simulink model "snap2_f_200msps_64i_4096c"  (R2019a)
settings: Solver=VariableStepDiscrete  StartTime=0.0  StopTime=10.0  RelTol=1e-3
undefined symbols (not defined in the file or in its folder): datetime, posixtime
libraries: xbsIndex_r4 x21354, casper_library_misc x297, casper_library_delays x19, xps_library x14, casper_library_sources x4
(part 13 of 217)

== system snap2_f_200msps_64i_4096c/cosmic_ray/Subsystem1 ==
  Constant24 : xbsIndex_r4/Constant  const=1  gui_display_data_type=Boolean  arith_type=Boolean  n_bits=1  bin_pt=0  preci_type=Single  exp_width=8  frac_width=24  explicit_period=on  period=1  equ=P=C  opselect=C  inp2=PCIN>>17  opr=+  inp1=P  carry=CIN  dbl_ovrd=off  block_type=constant
  Convert5 : xbsIndex_r4/Convert  gui_display_data_type=Boolean  arith_type=Boolean  n_bits=16  bin_pt=14  float_type=Single  exp_bits=8  fraction_bits=24  quantization=Truncate  overflow=Wrap  en=off  latency=1  pipeline=off  dbl_ovrd=off  block_type=convert
  Delay15 : xbsIndex_r4/Delay  rst=off  infoeditControl=Selection of Reset will increase slice count due to use of real FFs and instead of SRLs  en=off  latency=5000  reg_retiming=on  dbl_ovrd=off  block_type=delay
  Inverter5 : xbsIndex_r4/Inverter  en=off  latency=1  dbl_ovrd=off  block_type=inv
  Logical6 : xbsIndex_r4/Logical  logical_function=AND  inputs=2  en=off  latency=1  precision=Full  arith_type=Unsigned  n_bits=16  bin_pt=0  align_bp=on  dbl_ovrd=off  block_type=logical
  Slice22 : xbsIndex_r4/Slice  nbits=1  boolean_output=off  mode=Upper Bit Location + Width  bit1=0  base1=MSB of Input  bit0=0  base0=LSB of Input  dbl_ovrd=off  block_type=slice
  edge_detect4 : Subsystem  AncestorBlock=casper_library_misc/edge_detect  mask(edge_detect){edge=Rising, polarity=Active High, x_in=[0 0.08 0.08 0.16 0.16 0.24 0.24 0.32 0.32 0.4], y_in=[-1 -1  1  1  1  1  1  1  1  1], x_out=[0.6 0.68 0.68 0.76 0.76 0.84 0.84 0.92 0.92 1], y_out=[-1 -1  1  1 -1 -1 -1 -1 -1 -1]}
      mask prompts: edge "Edge Type"; polarity "Output Polarity"; x_in "Input X Positions"; y_in "Input Y Positions"; x_out "Output X Positions"; y_out "Output Y Positions"
      mask help: Output is active for one-cycle after each edge of the specified type (i.e. rising, falling or both).
      mask init: same as snap2_f_200msps_64i_4096c/cosmic_ray/edge_detect
      settings: AttributesFormatString=|
      | rising edges
      | active high
      mask Help: Output is active for one-cycle after each edge of the specified type (i.e. rising, falling, or both).  Latency is zero.
      mask TypeOptions edge: Rising | Falling | Both
      mask TypeOptions polarity: Active High | Active Low
      mask Display:
      | plot(x_in_num,0.5+y_in_num*0.2);
      | plot(x_out_num,0.5+y_out_num*0.2);
  trigger_sim5 : xbsIndex_r4/Counter  cnt_type=Free Running  cnt_to=1  operation=Up  start_count=1  cnt_by_val=1  arith_type=Unsigned  n_bits=3  bin_pt=0  load_pin=off  rst=off  en=on  explicit_period=off  period=1  use_behavioral_HDL=off  implementation=Fabric  dbl_ovrd=off  block_type=counter
  Out1 : Outport
  wires:
  Convert5/1 -> edge_detect4/1(in), Inverter5/1
  Slice22/1 -> Convert5/1
  Constant24/1 -> Logical6/2
  Delay15/1 -> Out1/1
  trigger_sim5/1 -> Slice22/1
  Logical6/1 -> trigger_sim5/1
  Inverter5/1 -> Logical6/1
  edge_detect4/1(out) -> Delay15/1

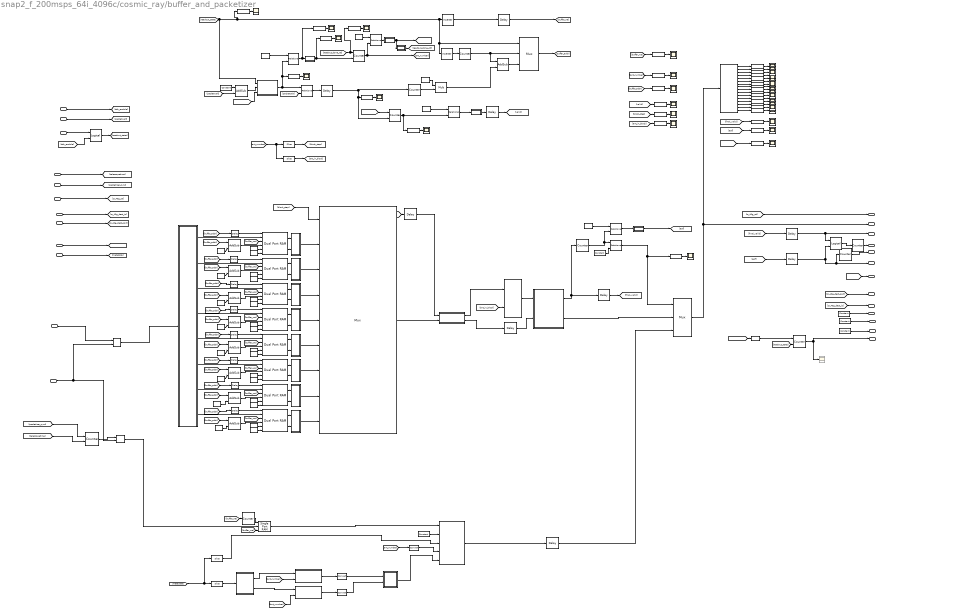
== system snap2_f_200msps_64i_4096c/cosmic_ray/buffer_and_packetizer ==
  note: The buffers' input is delayed is delayed in order to position the pulse in the middle of the buffer. The timestamp and data are delayed by the same amount.
  note: When load goes high, the counter takes the value provided by din, and then resumes counting up from there. Telescopetime is from tt_sync from the main design, which is the time of the last system sync expressed as unix time in number of clock cycles.
  note: Some delay here is needed to account for the time it takes the data to go through the rest of the packetizer. Probably a shorter delay around 20 clock cycles would suffice, but since the header only changes between packets, there shouldn't be any problem making it longer to be safe.
  note: The antenna counter increments whenever the main packet cycle counter falls back to zero. The readout is finished when the 6 bit antenna counter falls back to zero. Note that the last packet will be sent some (probably ~16) clock cycles after the readout done signal goes to 1, because it takes some time for the last data that is already on the way to make it through the packetizer.
  note: Note this works well in this situation where enable is high for a block of consecutive clock cycles. In other situations, it might have a limit that is up to 2 cycles lower. (So if copying this block to another design, test it).
  note: EOF and Valid both have a delay for the last mux on the data.
  note: 3 delay for counter, comparator and edge dectect above.
  note: Delay of 3 to account for buffer, mux, and delay on buffer address.
  note: 3 delays for valid to sync with buffer_addr during readout.
  note: Valid happens every 8 clock cycles.
  note: This counts to 2048 not 4096 because the address will increment in steps of two and both ports will be used to read out the buffer twice as fast as it was written.
  note: Data is buffered in dual-port BRAMs. Each of 8 BRAMS buffers 8 antennas bussed together. When writing data, the port A address continuesly increments by one on every clock cycle, as a circular buffer. Data input to port B is never enabled. When reading out data, both ports are used. Both addresses increment in steps of 2 and one port reads out odd time samples while the other reads out even samples. Both outputs are bussed together in order for the demux block to select the block of antennas that is currently being packetized.
  note: This block debusses the buffer output and then busses together adjacent pairs of samples from the same antenna and then does an 8x8 square transpose whose output on each clock cycle is 8 pairs of samples (total 16 consecutive samples) for one antenna. Every successive clock cycle is the next antenna, with the antenna repeating every 8 clock cycles.
  note: This mux increments which block of antennas to read out.
  note: Every valid increments the counter, which counts how many words have gone into the packet. Whenever the 8-bit counter loops back to zero, the packet header is inserted by the last mux below.
  note: End of frame occurs when the word counter resets.
  note: This mux chooses whether to send data or the header. The header is sent whenever the word count is zero-- i.e. the first word of the packet.
  note: Number of clock cycles spent in readout state.
  note: Signals that are only needed if receiving ethernet packets and thus are tied to zero in this design.
  note: Specifies the destination port and is controlled by a software register.
  note: Counters to track the number of eofs and eof+valid (which should be the number of packets). Eof must always occur on the last clock cycle where valid=1 for that packet, and so the eof counter and the eof+valid counter should match. Both are included for debugging purposes, as a common reason for not getting packets is when eof and valid misalign.
  note: Reset the ethernet port. This is tied to a software register.
  note: Data entering the ethernet block on clock cycles when valid=1 will go in the current packet.
  note: Data that will be clocked into the ethernet block whenever valid=1.
  note: End of frame to signify to the ethernet block that that the packet is ready.
  note: Readout is finished when eof occurs and the antenna number is 63.
  note: This is the packet header.
  note: convert to 8
  note: 3b
  note: 64b
  note: The timestamp buffer is write enabled whenever the data buffer is, but instead of reading out the whole timestamp buffer as is done for the data, the timestamp address stays fixed during readout at the place that it stopped writing. DOES THIS MEAN THAT THE TRANSMITTED TIMESTAMP IS THE OLDEST OR NEWEST IN THE BUFFER? It will be important to verify that the buffer address stops and restarts at the same address, and that this address is the same for the timestamp buffer and the data buffers.
  note: The upper three bits of the antenna number determine which block of 8 antennas is being packetized and the lower three bits determine which antenna within the block. These should increment during the wait between packets, so that the exact synchronization is less strict. However, if the delay through the other parts of the system is longer than packetwait, more careful delays on these signals may be needed.
  note: Wait for the software-tunable time between packets and then readout the buffer by cycling through addresses in steps of two, with odd and even being read out on the two different ports.
  note: Increment the buffer address by 1 whenever not in readout state, and by 2 when it's time to read out the buffer.
  note: Enable writing to the buffer whenever not in readout state. The delay of 3 is to sync up with the address when in listening state.
  note: Info to go in the packets saying if the trigger originated on this board, giving the board id, and saving the settings for the thresholds, windows, and roles.
  note: Counter number of clock cycles that the board spends in readout state during readout.
  note: Enable the timer while the board is in readout_state, reset from software.
  note: Specifies the destination ip and is controlled by a software register.
  note: This mux increments which antenna within the current block of antennas to read out. Out of the transpose block, every antenna repeats every 8 clock cycles. Single-antenna packets will be made by clocking data into the ethernet buffer once every 8 cycles. The choice of antenna is made by choosing between 8 different delay offsets on the sync signal, such that the valid is delayed according to which is chosen.
  pkt_wait : Inport
  tt : Inport  Port=2
  sync_in : Inport  Port=3
  eth40g_rst : Inport  Port=4
  dest_ip : Inport  Port=5
  dest_port : Inport  Port=6
  readout_timer_rst : Inport  Port=7
  data_in : Inport  Port=8
  readout_state : Inport  Port=9
  eth_enable : Inport  Port=10
  metadata : Inport  Port=11
  delay_buffer : Inport  Port=12
  AddSub : xbsIndex_r4/AddSub  mode=Addition  use_carryin=off  use_carryout=off  en=off  latency=1  precision=Full  arith_type=Unsigned  n_bits=16  bin_pt=14  quantization=Truncate  overflow=Wrap  use_behavioral_HDL=off  hw_selection=Fabric  pipelined=off  dbl_ovrd=off  block_type=addsub
  AddSub{1..9} (9 alike) : xbsIndex_r4/AddSub  mode=Addition  use_carryin=off  use_carryout=off  en=off  latency=1  precision=User Defined  arith_type=Unsigned  n_bits=12  bin_pt=0  quantization=Truncate  overflow=Wrap  use_behavioral_HDL=off  hw_selection=Fabric  pipelined=off  dbl_ovrd=off  block_type=addsub
  Constant : xbsIndex_r4/Constant  const=0  gui_display_data_type=Fixed-point  arith_type=Signed (2's comp)  n_bits=40  bin_pt=0  preci_type=Single  exp_width=8  frac_width=24  explicit_period=off  period=1  equ=P=C  opselect=C  inp2=PCIN>>17  opr=+  inp1=P  carry=CIN  dbl_ovrd=off  block_type=constant
  Constant{1,3..4,25} (4 alike) : xbsIndex_r4/Constant  const=0  gui_display_data_type=Fixed-point  arith_type=Unsigned  n_bits=3  bin_pt=0  preci_type=Single  exp_width=8  frac_width=24  explicit_period=on  period=1  equ=P=C  opselect=C  inp2=PCIN>>17  opr=+  inp1=P  carry=CIN  dbl_ovrd=off  block_type=constant
  Constant{6,8,10,12,14,16,18,20} (8 alike) : xbsIndex_r4/Constant  const=0  gui_display_data_type=Fixed-point  arith_type=Unsigned  n_bits=80  bin_pt=0  preci_type=Single  exp_width=8  frac_width=24  explicit_period=on  period=1  equ=P=C  opselect=C  inp2=PCIN>>17  opr=+  inp1=P  carry=CIN  dbl_ovrd=off  block_type=constant
  Constant{7,9,11,13,15,17,19,21} (8 alike) : xbsIndex_r4/Constant  const=0  gui_display_data_type=Boolean  arith_type=Boolean  n_bits=1  bin_pt=0  preci_type=Single  exp_width=8  frac_width=24  explicit_period=on  period=1  equ=P=C  opselect=C  inp2=PCIN>>17  opr=+  inp1=P  carry=CIN  dbl_ovrd=off  block_type=constant
  Constant{2,26..27,29..32,34} (8 alike) : xbsIndex_r4/Constant  const=1  gui_display_data_type=Fixed-point  arith_type=Unsigned  n_bits=1  bin_pt=0  preci_type=Single  exp_width=8  frac_width=24  explicit_period=on  period=1  equ=P=C  opselect=C  inp2=PCIN>>17  opr=+  inp1=P  carry=CIN  dbl_ovrd=off  block_type=constant
  Constant22 : xbsIndex_r4/Constant  const=0  gui_display_data_type=Boolean  arith_type=Boolean  n_bits=16  bin_pt=14  preci_type=Single  exp_width=8  frac_width=24  explicit_period=on  period=1  equ=P=C  opselect=C  inp2=PCIN>>17  opr=+  inp1=P  carry=CIN  dbl_ovrd=off  block_type=constant
  Constant23 : xbsIndex_r4/Constant  const=0  gui_display_data_type=Boolean  arith_type=Boolean  n_bits=16  bin_pt=14  preci_type=Single  exp_width=8  frac_width=24  explicit_period=on  period=1  equ=P=C  opselect=C  inp2=PCIN>>17  opr=+  inp1=P  carry=CIN  dbl_ovrd=off  block_type=constant
  Constant24 : xbsIndex_r4/Constant  const=2  gui_display_data_type=Fixed-point  arith_type=Unsigned  n_bits=2  bin_pt=0  preci_type=Single  exp_width=8  frac_width=24  explicit_period=on  period=1  equ=P=C  opselect=C  inp2=PCIN>>17  opr=+  inp1=P  carry=CIN  dbl_ovrd=off  block_type=constant
  Constant28 : xbsIndex_r4/Constant  const=0  gui_display_data_type=Boolean  arith_type=Boolean  n_bits=16  bin_pt=14  preci_type=Single  exp_width=8  frac_width=24  explicit_period=on  period=1  equ=P=C  opselect=C  inp2=PCIN>>17  opr=+  inp1=P  carry=CIN  dbl_ovrd=off  block_type=constant
  Constant33 : xbsIndex_r4/Constant  const=2048  gui_display_data_type=Fixed-point  arith_type=Unsigned  n_bits=12  bin_pt=0  preci_type=Single  exp_width=8  frac_width=24  explicit_period=on  period=1  equ=P=C  opselect=C  inp2=PCIN>>17  opr=+  inp1=P  carry=CIN  dbl_ovrd=off  block_type=constant
  Constant5 : xbsIndex_r4/Constant  const=0  gui_display_data_type=Fixed-point  arith_type=Unsigned  n_bits=8  bin_pt=0  preci_type=Single  exp_width=8  frac_width=24  explicit_period=on  period=1  equ=P=C  opselect=C  inp2=PCIN>>17  opr=+  inp1=P  carry=CIN  dbl_ovrd=off  block_type=constant
  Convert1 : xbsIndex_r4/Convert  gui_display_data_type=Fixed-point  arith_type=Unsigned  n_bits=8  bin_pt=0  float_type=Single  exp_bits=8  fraction_bits=24  quantization=Truncate  overflow=Wrap  en=off  latency=1  pipeline=off  dbl_ovrd=off  block_type=convert
  Convert2 : xbsIndex_r4/Convert  gui_display_data_type=Fixed-point  arith_type=Unsigned  n_bits=8  bin_pt=0  float_type=Single  exp_bits=8  fraction_bits=24  quantization=Truncate  overflow=Wrap  en=off  latency=1  pipeline=off  dbl_ovrd=off  block_type=convert
  Convert3 : xbsIndex_r4/Convert  gui_display_data_type=Fixed-point  arith_type=Unsigned  n_bits=8  bin_pt=0  float_type=Single  exp_bits=8  fraction_bits=24  quantization=Truncate  overflow=Wrap  en=off  latency=1  pipeline=off  dbl_ovrd=off  block_type=convert
  Counter2 : xbsIndex_r4/Counter  cnt_type=Free Running  cnt_to=Inf  operation=Up  start_count=0  cnt_by_val=1  arith_type=Unsigned  n_bits=32  bin_pt=0  load_pin=off  rst=off  en=on  explicit_period=on  period=1  use_behavioral_HDL=off  implementation=Fabric  dbl_ovrd=off  block_type=counter
  Counter5 : xbsIndex_r4/Counter  cnt_type=Free Running  cnt_to=Inf  operation=Up  start_count=0  cnt_by_val=1  arith_type=Unsigned  n_bits=32  bin_pt=0  load_pin=off  rst=off  en=on  explicit_period=on  period=1  use_behavioral_HDL=off  implementation=Fabric  dbl_ovrd=off  block_type=counter
  Delay1 : xbsIndex_r4/Delay  rst=off  infoeditControl=Selection of Reset will increase slice count due to use of real FFs and instead of SRLs  en=off  latency=3  reg_retiming=off  dbl_ovrd=off  block_type=delay
  Delay{2,4..10,12,14,16} (11 alike) : xbsIndex_r4/Delay  rst=off  infoeditControl=Selection of Reset will increase slice count due to use of real FFs and instead of SRLs  en=off  latency=1  reg_retiming=off  dbl_ovrd=off  block_type=delay
  Delay11 : xbsIndex_r4/Delay  rst=off  infoeditControl=Selection of Reset will increase slice count due to use of real FFs and instead of SRLs  en=off  latency=3  reg_retiming=off  dbl_ovrd=off  block_type=delay
  Delay13 : xbsIndex_r4/Delay  rst=off  infoeditControl=Selection of Reset will increase slice count due to use of real FFs and instead of SRLs  en=off  latency=2  reg_retiming=off  dbl_ovrd=off  block_type=delay
  Delay17 : xbsIndex_r4/Delay  rst=off  infoeditControl=Selection of Reset will increase slice count due to use of real FFs and instead of SRLs  en=off  latency=128  reg_retiming=off  dbl_ovrd=off  block_type=delay
  Delay24 : xbsIndex_r4/Delay  rst=off  infoeditControl=Selection of Reset will increase slice count due to use of real FFs and instead of SRLs  en=off  latency=1  reg_retiming=on  dbl_ovrd=off  block_type=delay
  Delay3 : xbsIndex_r4/Delay  rst=off  infoeditControl=Selection of Reset will increase slice count due to use of real FFs and instead of SRLs  en=off  latency=3  reg_retiming=off  dbl_ovrd=off  block_type=delay
  Dual Port RAM{,1..7} (8 alike) : xbsIndex_r4/Dual Port RAM  depth=4096  initVector=sin(pi*(0:15)/16)  distributed_mem=Block RAM  init_a=0  init_b=0  rst_a=off  rst_b=off  en_a=off  en_b=off  latency=1  write_mode_A=Read After Write  write_mode_B=Read After Write  optimize=Area  dbl_ovrd=off  block_type=dpram
  Gateway Out{2..34} (33 alike) : xbsIndex_r4/Gateway Out  inherit_from_input=off  hdl_port=on  rows=1  columns=1  UseAsDAC=off  DACChannel='1'  interface=None  automatic_assignment=on  address_offset=hex2dec('00')  intf_name=''  intf_description=''  timing_constraint=None  locs_specified=off  LOCs={}  io_standard={}  block_type=gatewayout
  Inverter : xbsIndex_r4/Inverter  en=off  latency=1  dbl_ovrd=off  block_type=inv
  Inverter1 : xbsIndex_r4/Inverter  en=off  latency=1  dbl_ovrd=off  block_type=inv
  Logical : xbsIndex_r4/Logical  logical_function=AND  inputs=2  en=off  latency=1  precision=Full  arith_type=Unsigned  n_bits=16  bin_pt=0  align_bp=on  dbl_ovrd=off  block_type=logical
  Logical3 : xbsIndex_r4/Logical  logical_function=AND  inputs=2  en=off  latency=1  precision=Full  arith_type=Unsigned  n_bits=16  bin_pt=0  align_bp=on  dbl_ovrd=off  block_type=logical
  Mult : xbsIndex_r4/Mult  precision=Full  arith_type="Signed  (2's comp)"  n_bits=16  bin_pt=14  quantization=Truncate  overflow=Wrap  en=off  latency=3  use_behavioral_HDL=off  opt=Speed  use_embedded=on  optimum_pipeline=off  pipeline=on  dbl_ovrd=off  use_rpm=on  placement_style=Triangular  block_type=mult
  Mux1 : xbsIndex_r4/Mux  inputs=2  en=off  latency=1  precision=Full  arith_type=Unsigned  n_bits=16  bin_pt=14  quantization=Truncate  overflow=Wrap  dbl_ovrd=off  block_type=mux
  Mux2 : xbsIndex_r4/Mux  inputs=8  en=off  latency=1  precision=Full  arith_type=Unsigned  n_bits=16  bin_pt=14  quantization=Truncate  overflow=Wrap  dbl_ovrd=off  block_type=mux
  Mux4 : xbsIndex_r4/Mux  inputs=2  en=off  latency=1  precision=Full  arith_type=Unsigned  n_bits=16  bin_pt=14  quantization=Truncate  overflow=Wrap  dbl_ovrd=off  block_type=mux
  Relational{1,4..5,7} (4 alike) : xbsIndex_r4/Relational  mode=a<b  op_type=Bool  en=off  latency=1  dbl_ovrd=off  block_type=relational
  Relational2 : xbsIndex_r4/Relational  mode=a>b  op_type=Bool  en=off  latency=1  dbl_ovrd=off  block_type=relational
  Relational6 : xbsIndex_r4/Relational  mode=a=b  op_type=Bool  en=off  latency=1  dbl_ovrd=off  block_type=relational
  Scope{,1..14,16..33} (33 alike) : Scope
  Scope15 : Scope  Commented=on
  Single Port RAM1 : xbsIndex_r4/Single Port RAM  depth=4096  initVector=sin(pi*(0:15)/16)  distributed_mem=Block RAM  write_mode=Read After Write  rst=off  init_reg=0  en=off  latency=1  optimize=Speed  dbl_ovrd=off  block_type=spram
  Subsystem1 : Subsystem
  Subsystem2 : Subsystem
  antenna_counter : xbsIndex_r4/Counter  cnt_type=Free Running  cnt_to=1  operation=Up  start_count=0  cnt_by_val=1  arith_type=Unsigned  n_bits=6  bin_pt=0  load_pin=off  rst=on  en=on  explicit_period=off  period=1  use_behavioral_HDL=off  implementation=Fabric  dbl_ovrd=off  block_type=counter
  buffer_addr : xbsIndex_r4/Counter  cnt_type=Free Running  cnt_to=1  operation=Up  start_count=0  cnt_by_val=1  arith_type=Unsigned  n_bits=11  bin_pt=0  load_pin=off  rst=off  en=on  explicit_period=off  period=1  use_behavioral_HDL=off  implementation=Fabric  dbl_ovrd=off  block_type=counter
  buffer_addr2 : xbsIndex_r4/Counter  cnt_type=Free Running  cnt_to=1  operation=Up  start_count=0  cnt_by_val=1  arith_type=Unsigned  n_bits=12  bin_pt=0  load_pin=off  rst=off  en=on  explicit_period=off  period=1  use_behavioral_HDL=off  implementation=Fabric  dbl_ovrd=off  block_type=counter
  buffer_start_addr : xbsIndex_r4/Counter  cnt_type=Free Running  cnt_to=1  operation=Up  start_count=0  cnt_by_val=1  arith_type=Unsigned  n_bits=12  bin_pt=0  load_pin=off  rst=off  en=on  explicit_period=off  period=1  use_behavioral_HDL=off  implementation=Fabric  dbl_ovrd=off  block_type=counter
  bus-convert-16b : Subsystem
  bus_create1 : Subsystem  AncestorBlock=casper_library_flow_control/bus_create  mask(bus_create){inputNum=2}
      mask prompts: inputNum "Number of inputs:"
      mask init:
      | bus_create_init(gcb,...
      |     'inputNum', inputNum);
  bus_create10 : Subsystem  AncestorBlock=casper_library_flow_control/bus_create  mask(bus_create){inputNum=2}
      mask prompts: inputNum "Number of inputs:"
      mask init:
      | bus_create_init(gcb,...
      |     'inputNum', inputNum);
  bus_create2 : Subsystem  AncestorBlock=casper_library_flow_control/bus_create  mask(bus_create){inputNum=2}
      mask prompts: inputNum "Number of inputs:"
      mask init:
      | bus_create_init(gcb,...
      |     'inputNum', inputNum);
  bus_create3 : Subsystem  AncestorBlock=casper_library_flow_control/bus_create  mask(bus_create){inputNum=2}
      mask prompts: inputNum "Number of inputs:"
      mask init:
      | bus_create_init(gcb,...
      |     'inputNum', inputNum);
  bus_create4 : Subsystem  AncestorBlock=casper_library_flow_control/bus_create  mask(bus_create){inputNum=5}
      mask prompts: inputNum "Number of inputs:"
      mask init:
      | bus_create_init(gcb,...
      |     'inputNum', inputNum);
  bus_create5 : Subsystem  AncestorBlock=casper_library_flow_control/bus_create  mask(bus_create){inputNum=2}
      mask prompts: inputNum "Number of inputs:"
      mask init:
      | bus_create_init(gcb,...
      |     'inputNum', inputNum);
  bus_create6 : Subsystem  AncestorBlock=casper_library_flow_control/bus_create  mask(bus_create){inputNum=2}
      mask prompts: inputNum "Number of inputs:"
      mask init:
      | bus_create_init(gcb,...
      |     'inputNum', inputNum);
  bus_create7 : Subsystem  AncestorBlock=casper_library_flow_control/bus_create  mask(bus_create){inputNum=2}
      mask prompts: inputNum "Number of inputs:"
      mask init:
      | bus_create_init(gcb,...
      |     'inputNum', inputNum);
  bus_create8 : Subsystem  AncestorBlock=casper_library_flow_control/bus_create  mask(bus_create){inputNum=2}
      mask prompts: inputNum "Number of inputs:"
      mask init:
      | bus_create_init(gcb,...
      |     'inputNum', inputNum);
  bus_create9 : Subsystem  AncestorBlock=casper_library_flow_control/bus_create  mask(bus_create){inputNum=2}
      mask prompts: inputNum "Number of inputs:"
      mask init:
      | bus_create_init(gcb,...
      |     'inputNum', inputNum);
  bus_expand1 : Subsystem  AncestorBlock=casper_library_flow_control/bus_expand  mask(bus_expand){mode=divisions of equal size, outputNum=8, outputWidth=80, outputBinaryPt=0, outputArithmeticType=0, show_format=off, outputToWorkspace=off, variablePrefix=out, outputToModelAsWell=on}
      mask prompts: outputNum "Number of outputs:"; outputWidth "Output width:"; outputBinaryPt "Output binary point position:"; outputArithmeticType "Output arithmetic type (ufix=0, fix=1, bool=2):"; show_format "Print format string?"; outputToWorkspace "Output to workspace?"; variablePrefix "Variable name prefix:"; outputToModelAsWell "Output to model as well?"
      mask help:
      | Expands a 'bus' made using a bus_create or Xilinx
      | concat block.
      | The input will be divided into the specified number
      | of outputs with the specified arithmetic types.
      | Divisions are made from most significant bit.
      mask init: same as snap2_f_200msps_64i_4096c/autocorr/bus_expand
      settings: AttributesFormatString=8 outputs
      mask TypeOptions mode: divisions of equal size | divisions of arbitrary size
      mask Callback mode: bus_expand_callback();
      mask Callback outputWidth: bus_expand_callback();
      mask Callback outputToWorkspace: bus_expand_callback();
  bus_expand2 : Subsystem  AncestorBlock=casper_library_flow_control/bus_expand  mask(bus_expand){mode=divisions of equal size, outputNum=2, outputWidth=64, outputBinaryPt=0, outputArithmeticType=0, show_format=off, outputToWorkspace=off, variablePrefix=out, outputToModelAsWell=on}
      mask prompts: outputNum "Number of outputs:"; outputWidth "Output width:"; outputBinaryPt "Output binary point position:"; outputArithmeticType "Output arithmetic type (ufix=0, fix=1, bool=2):"; show_format "Print format string?"; outputToWorkspace "Output to workspace?"; variablePrefix "Variable name prefix:"; outputToModelAsWell "Output to model as well?"
      mask help:
      | Expands a 'bus' made using a bus_create or Xilinx
      | concat block.
      | The input will be divided into the specified number
      | of outputs with the specified arithmetic types.
      | Divisions are made from most significant bit.
      mask init: same as snap2_f_200msps_64i_4096c/autocorr/bus_expand
      settings: AttributesFormatString=2 outputs
      mask TypeOptions mode: divisions of equal size | divisions of arbitrary size
      mask Callback mode: bus_expand_callback();
      mask Callback outputWidth: bus_expand_callback();
      mask Callback outputToWorkspace: bus_expand_callback();
  bus_expand3 : Subsystem  AncestorBlock=casper_library_flow_control/bus_expand  mask(bus_expand){mode=divisions of equal size, outputNum=16, outputWidth=16, outputBinaryPt=0, outputArithmeticType=1, show_format=off, outputToWorkspace=off, variablePrefix=out, outputToModelAsWell=on}
      mask prompts: outputNum "Number of outputs:"; outputWidth "Output width:"; outputBinaryPt "Output binary point position:"; outputArithmeticType "Output arithmetic type (ufix=0, fix=1, bool=2):"; show_format "Print format string?"; outputToWorkspace "Output to workspace?"; variablePrefix "Variable name prefix:"; outputToModelAsWell "Output to model as well?"
      mask help:
      | Expands a 'bus' made using a bus_create or Xilinx
      | concat block.
      | The input will be divided into the specified number
      | of outputs with the specified arithmetic types.
      | Divisions are made from most significant bit.
      mask init: same as snap2_f_200msps_64i_4096c/autocorr/bus_expand
      settings: AttributesFormatString=16 outputs
      mask TypeOptions mode: divisions of equal size | divisions of arbitrary size
      mask Callback mode: bus_expand_callback();
      mask Callback outputWidth: bus_expand_callback();
      mask Callback outputToWorkspace: bus_expand_callback();
  count-limited-counter : Subsystem
  count-to-8 : xbsIndex_r4/Counter  cnt_type=Free Running  cnt_to=1  operation=Up  start_count=0  cnt_by_val=1  arith_type=Unsigned  n_bits=3  bin_pt=0  load_pin=off  rst=on  en=on  explicit_period=off  period=1  use_behavioral_HDL=off  implementation=Fabric  dbl_ovrd=off  block_type=counter
  count-words : xbsIndex_r4/Counter  cnt_type=Free Running  cnt_to=1  operation=Up  start_count=0  cnt_by_val=1  arith_type=Unsigned  n_bits=8  bin_pt=0  load_pin=off  rst=off  en=on  explicit_period=off  period=1  use_behavioral_HDL=off  implementation=Fabric  dbl_ovrd=off  block_type=counter
  delay_bram_prog1 : casper_library_delays/delay_bram_prog  MaxDelay=7  bram_latency=4
      settings: SourceProductName=CASPER DSP Blockset
  delay_bram_prog2 : casper_library_delays/delay_bram_prog  MaxDelay=7  bram_latency=4
      settings: SourceProductName=CASPER DSP Blockset
  edge_detect1 : Subsystem  AncestorBlock=casper_library_misc/edge_detect  mask(edge_detect){edge=Falling, polarity=Active High, x_in=[0 0.08 0.08 0.16 0.16 0.24 0.24 0.32 0.32 0.4], y_in=[-1 -1  1  1  1  1  1  1  1  1], x_out=[0.6 0.68 0.68 0.76 0.76 0.84 0.84 0.92 0.92 1], y_out=[-1 -1  1  1 -1 -1 -1 -1 -1 -1]}
      mask prompts: edge "Edge Type"; polarity "Output Polarity"; x_in "Input X Positions"; y_in "Input Y Positions"; x_out "Output X Positions"; y_out "Output Y Positions"
      mask help: Output is active for one-cycle after each edge of the specified type (i.e. rising, falling or both).
      mask init: same as snap2_f_200msps_64i_4096c/cosmic_ray/edge_detect
      settings: AttributesFormatString=|
      | falling edges
      | active high
      mask Help: Output is active for one-cycle after each edge of the specified type (i.e. rising, falling, or both).  Latency is zero.
      mask TypeOptions edge: Rising | Falling | Both
      mask TypeOptions polarity: Active High | Active Low
      mask Display:
      | plot(x_in_num,0.5+y_in_num*0.2);
      | plot(x_out_num,0.5+y_out_num*0.2);
  edge_detect15 : casper_library_misc/edge_detect  edge=Rising  polarity=Active High  x_in=[0 0.08 0.08 0.16 0.16 0.24 0.24 0.32 0.32 0.4]  y_in="[-1 -1  1  1  1  1  1  1  1  1]"  x_out=[0.6 0.68 0.68 0.76 0.76 0.84 0.84 0.92 0.92 1]  y_out="[-1 -1  1  1 -1 -1 -1 -1 -1 -1]"
  edge_detect2 : Subsystem  AncestorBlock=casper_library_misc/edge_detect  mask(edge_detect){edge=Falling, polarity=Active High, x_in=[0 0.08 0.08 0.16 0.16 0.24 0.24 0.32 0.32 0.4], y_in=[-1 -1  1  1  1  1  1  1  1  1], x_out=[0.6 0.68 0.68 0.76 0.76 0.84 0.84 0.92 0.92 1], y_out=[-1 -1  1  1 -1 -1 -1 -1 -1 -1]}
      mask prompts: edge "Edge Type"; polarity "Output Polarity"; x_in "Input X Positions"; y_in "Input Y Positions"; x_out "Output X Positions"; y_out "Output Y Positions"
      mask help: Output is active for one-cycle after each edge of the specified type (i.e. rising, falling or both).
      mask init: same as snap2_f_200msps_64i_4096c/cosmic_ray/edge_detect
      settings: AttributesFormatString=|
      | falling edges
      | active high
      mask Help: Output is active for one-cycle after each edge of the specified type (i.e. rising, falling, or both).  Latency is zero.
      mask TypeOptions edge: Rising | Falling | Both
      mask TypeOptions polarity: Active High | Active Low
      mask Display:
      | plot(x_in_num,0.5+y_in_num*0.2);
      | plot(x_out_num,0.5+y_out_num*0.2);
  edge_detect3 : Subsystem  AncestorBlock=casper_library_misc/edge_detect  mask(edge_detect){edge=Falling, polarity=Active High, x_in=[0 0.08 0.08 0.16 0.16 0.24 0.24 0.32 0.32 0.4], y_in=[-1 -1  1  1  1  1  1  1  1  1], x_out=[0.6 0.68 0.68 0.76 0.76 0.84 0.84 0.92 0.92 1], y_out=[-1 -1  1  1 -1 -1 -1 -1 -1 -1]}
      mask prompts: edge "Edge Type"; polarity "Output Polarity"; x_in "Input X Positions"; y_in "Input Y Positions"; x_out "Output X Positions"; y_out "Output Y Positions"
      mask help: Output is active for one-cycle after each edge of the specified type (i.e. rising, falling or both).
      mask init: same as snap2_f_200msps_64i_4096c/cosmic_ray/edge_detect
      settings: AttributesFormatString=|
      | falling edges
      | active high
      mask Help: Output is active for one-cycle after each edge of the specified type (i.e. rising, falling, or both).  Latency is zero.
      mask TypeOptions edge: Rising | Falling | Both
      mask TypeOptions polarity: Active High | Active Low
      mask Display:
      | plot(x_in_num,0.5+y_in_num*0.2);
      | plot(x_out_num,0.5+y_out_num*0.2);
  edge_detect4 : Subsystem  AncestorBlock=casper_library_misc/edge_detect  mask(edge_detect){edge=Falling, polarity=Active High, x_in=[0 0.08 0.08 0.16 0.16 0.24 0.24 0.32 0.32 0.4], y_in=[-1 -1  1  1  1  1  1  1  1  1], x_out=[0.6 0.68 0.68 0.76 0.76 0.84 0.84 0.92 0.92 1], y_out=[-1 -1  1  1 -1 -1 -1 -1 -1 -1]}
      mask prompts: edge "Edge Type"; polarity "Output Polarity"; x_in "Input X Positions"; y_in "Input Y Positions"; x_out "Output X Positions"; y_out "Output Y Positions"
      mask help: Output is active for one-cycle after each edge of the specified type (i.e. rising, falling or both).
      mask init: same as snap2_f_200msps_64i_4096c/cosmic_ray/edge_detect
      settings: AttributesFormatString=|
      | falling edges
      | active high
      mask Help: Output is active for one-cycle after each edge of the specified type (i.e. rising, falling, or both).  Latency is zero.
      mask TypeOptions edge: Rising | Falling | Both
      mask TypeOptions polarity: Active High | Active Low
      mask Display:
      | plot(x_in_num,0.5+y_in_num*0.2);
      | plot(x_out_num,0.5+y_out_num*0.2);
  lower3bits : xbsIndex_r4/Slice  nbits=3  boolean_output=off  mode=Lower Bit Location + Width  bit1=0  base1=MSB of Input  bit0=0  base0=LSB of Input  dbl_ovrd=off  block_type=slice
  pulse_ext : Subsystem  AncestorBlock=casper_library_misc/pulse_ext  mask(pulse_ext){pulse_len=32}
      mask prompts: pulse_len "Length of Pulse"
      mask help:
      | Extends a boolean signal to be high for the specified number of clocks after
      | the last high input.
      mask init:
      | bits = ceil(log2(pulse_len+1));
      mask Help: eval('xlWeb(''http://casper.berkeley.edu/wiki/Pulse_ext'')')
  readout_timer1 : xbsIndex_r4/Counter  cnt_type=Free Running  cnt_to=1  operation=Up  start_count=0  cnt_by_val=1  arith_type=Unsigned  n_bits=32  bin_pt=0  load_pin=off  rst=on  en=on  explicit_period=off  period=1  use_behavioral_HDL=off  implementation=Fabric  dbl_ovrd=off  block_type=counter
  "select_antenna " : Subsystem
  slice : xbsIndex_r4/Slice  nbits=128  boolean_output=off  mode=Lower Bit Location + Width  bit1=0  base1=MSB of Input  bit0=0  base0=LSB of Input  dbl_ovrd=off  block_type=slice
  slice1 : xbsIndex_r4/Slice  nbits=128  boolean_output=off  mode=Upper Bit Location + Width  bit1=0  base1=MSB of Input  bit0=0  base0=LSB of Input  dbl_ovrd=off  block_type=slice
  transpose : Subsystem
  tt_counter : xbsIndex_r4/Counter  cnt_type=Free Running  cnt_to=1  operation=Up  start_count=0  cnt_by_val=1  arith_type=Unsigned  n_bits=64  bin_pt=0  load_pin=on  rst=off  en=off  explicit_period=on  period=1  use_behavioral_HDL=off  implementation=Fabric  use_rpm=on  dbl_ovrd=off  block_type=counter
      settings: xl_area=[0, 0, 0, 0, 0, 0, 0]
  upper3bits : xbsIndex_r4/Slice  nbits=3  boolean_output=off  mode=Upper Bit Location + Width  bit1=0  base1=MSB of Input  bit0=0  base0=LSB of Input  dbl_ovrd=off  block_type=slice
  eth40g_rst_out : Outport
  data_out : Outport  Port=2
  valid : Outport  Port=3
  dest_ip_40g : Outport  Port=4
  dest_port_40g : Outport  Port=5
  eof : Outport  Port=6
  zero_rx_signal : Outport  Port=7
  zero_rx_signal1 : Outport  Port=8
  zero_rx_signal2 : Outport  Port=9
  eof_ctr : Outport  Port=10
  eof_and_valid_ctr : Outport  Port=11
  "readout_timer " : Outport  Port=12
  "readout_done " : Outport  Port=13
  wires:
  [cr_40g_dest_ip] -> dest_ip_40g/1
  pkt_wait/1 -> [packetwait]
  Constant22/1 -> zero_rx_signal1/1
  [cr_40g_dest_port] -> dest_port_40g/1
  Constant23/1 -> zero_rx_signal/1
  Constant28/1 -> zero_rx_signal2/1
  tt/1 -> [telescopetime]
  sync_in/1 -> [packetizer_sync]
  readout_timer1/1 -> Scope15/1, "readout_timer "/1
  dest_ip/1 -> [cr_40g_dest_ip]
  eth40g_rst/1 -> [cr_40g_rst]
  dest_port/1 -> [cr_40g_dest_port]
  edge_detect15/1 -> readout_timer1/1
  [readout_timer_rst] -> edge_detect15/1
  readout_timer_rst/1 -> [readout_timer_rst]
  [readout_state] -> readout_timer1/2
  eth_enable/1 -> [eth_enable]
  [eth_enable] -> Logical/2
  Logical/1 -> [readout_state]
  readout_state/1 -> Logical/1
  metadata/1 -> [metadata]
  [buffer_we] -> Dual Port RAM/3
  [block_step] -> Mux2/1
  Delay11/1 -> transpose/1(sync_in)
  [eof] -> Delay14/1
  Logical3/1 -> Counter5/1
  [final_valid] -> Delay2/1
  Counter5/1 -> eof_and_valid_ctr/1
  Counter2/1 -> eof_ctr/1
  Inverter/1 -> Delay1/1
  Relational2/1 -> Delay16/1
  count-limited-counter/1(out) -> Relational4/2, Gateway Out29/1, Relational2/1
  AddSub/1 -> count-limited-counter/2(limit)
  [packetwait] -> AddSub/2
  [readout_state] -> count-limited-counter/1(en), Gateway Out30/1, Mux4/1, Inverter1/1, Inverter/1
  Constant33/1 -> AddSub/1
  Delay1/1 -> [buffer_we]
  antenna_counter/1 -> Relational1/2, [ant_number]
  [ant_number] -> lower3bits/1, upper3bits/1
  upper3bits/1 -> [block_step]
  lower3bits/1 -> [ant_in_block]
  [buffer_we] -> Single Port RAM1/3
  [buffer_we] -> buffer_addr2/1
  buffer_addr2/1 -> Single Port RAM1/1
  Single Port RAM1/1 -> bus_create4/1(in1)
  [ant_number] -> Convert2/1
  [metadata] -> slice1/1, slice/1
  bus_create1/1(bus_out) -> bus_create4/5(in5)
  Convert2/1 -> bus_create4/4(in4)
  slice/1 -> bus_expand2/1(bus_in)
  Convert1/1 -> bus_create1/1(in1)
  Convert3/1 -> bus_create1/2(in2)
  slice1/1 -> bus_create4/3(in3)
  bus_create4/1(bus_out) -> Delay17/1
  count-to-8/1 -> Gateway Out31/1, Relational7/2
  edge_detect3/1(out) -> Delay3/1
  count-words/1 -> Relational5/2, Relational6/1
  Mux1/1 -> data_out/1, bus_expand3/1(bus_in)
  Relational6/1 -> Mux1/1, Gateway Out8/1
  Delay2/1 -> valid/1, Logical3/1
  [ant_number] -> Subsystem1/2(antenna_number)
  Constant5/1 -> Relational6/2
  Subsystem1/1(Out1) -> Convert3/1
  bus_expand2/2(lsb_out1) -> Subsystem1/1(antenna_roles)
  Subsystem2/1(Out1) -> Convert1/1
  [ant_number] -> Subsystem2/2(antenna_number)
  bus_expand2/1(msb_out2) -> Subsystem2/1(antenna_roles)
  Constant6/1 -> Dual Port RAM/5
  Constant7/1 -> Dual Port RAM/6
  Delay4/1 -> Dual Port RAM/1
  bus-convert-16b/2(data_out) -> Mux1/2
  Dual Port RAM/1 -> bus_create2/1(in1)
  Dual Port RAM/2 -> bus_create2/2(in2)
  bus_create2/1(bus_out) -> Mux2/2
  Dual Port RAM1/2 -> bus_create3/2(in2)
  Dual Port RAM1/1 -> bus_create3/1(in1)
  Delay5/1 -> Dual Port RAM1/1
  Constant9/1 -> Dual Port RAM1/6
  Constant8/1 -> Dual Port RAM1/5
  [buffer_we] -> Dual Port RAM1/3
  [buffer_addr] -> Delay5/1
  [buffer_addr] -> Delay7/1
  [buffer_we] -> Dual Port RAM3/3
  Constant12/1 -> Dual Port RAM3/5
  Constant13/1 -> Dual Port RAM3/6
  Delay7/1 -> Dual Port RAM3/1
  Dual Port RAM3/1 -> bus_create6/1(in1)
  Dual Port RAM3/2 -> bus_create6/2(in2)
  Dual Port RAM2/2 -> bus_create5/2(in2)
  Dual Port RAM2/1 -> bus_create5/1(in1)
  Delay6/1 -> Dual Port RAM2/1
  Constant11/1 -> Dual Port RAM2/6
  Constant10/1 -> Dual Port RAM2/5
  [buffer_we] -> Dual Port RAM2/3
  [buffer_addr] -> Delay6/1
  [buffer_addr] -> Delay10/1
  [buffer_we] -> Dual Port RAM6/3
  Constant14/1 -> Dual Port RAM6/5
  Constant15/1 -> Dual Port RAM6/6
  Delay10/1 -> Dual Port RAM6/1
  Dual Port RAM6/1 -> bus_create9/1(in1)
  Dual Port RAM6/2 -> bus_create9/2(in2)
  Dual Port RAM7/2 -> bus_create10/2(in2)
  Dual Port RAM7/1 -> bus_create10/1(in1)
  Delay12/1 -> Dual Port RAM7/1
  Constant17/1 -> Dual Port RAM7/6
  Constant16/1 -> Dual Port RAM7/5
  [buffer_we] -> Dual Port RAM7/3
  [buffer_addr] -> Delay12/1
  [buffer_addr] -> Delay9/1
  [buffer_we] -> Dual Port RAM5/3
  Constant20/1 -> Dual Port RAM5/5
  Constant21/1 -> Dual Port RAM5/6
  Delay9/1 -> Dual Port RAM5/1
  Dual Port RAM5/1 -> bus_create8/1(in1)
  Dual Port RAM5/2 -> bus_create8/2(in2)
  Dual Port RAM4/2 -> bus_create7/2(in2)
  Dual Port RAM4/1 -> bus_create7/1(in1)
  Delay8/1 -> Dual Port RAM4/1
  Constant19/1 -> Dual Port RAM4/6
  Constant18/1 -> Dual Port RAM4/5
  [buffer_we] -> Dual Port RAM4/3
  [buffer_addr] -> Delay8/1
  bus_expand1/7(out2) -> Dual Port RAM6/2
  bus_expand1/8(lsb_out1) -> Dual Port RAM7/2
  bus_expand1/6(out3) -> Dual Port RAM5/2
  bus_expand1/5(out4) -> Dual Port RAM4/2
  bus_expand1/4(out5) -> Dual Port RAM3/2
  bus_expand1/3(out6) -> Dual Port RAM2/2
  bus_expand1/2(out7) -> Dual Port RAM1/2
  bus_expand1/1(msb_out8) -> Dual Port RAM/2
  bus_create3/1(bus_out) -> Mux2/3
  bus_create5/1(bus_out) -> Mux2/4
  bus_create6/1(bus_out) -> Mux2/5
  bus_create7/1(bus_out) -> Mux2/6
  bus_create8/1(bus_out) -> Mux2/7
  bus_create9/1(bus_out) -> Mux2/8
  bus_create10/1(bus_out) -> Mux2/9
  buffer_start_addr/1 -> AddSub1/1, Mux4/2
  Inverter1/1 -> buffer_start_addr/1
  Mux4/1 -> [buffer_addr]
  buffer_addr/1 -> Mult/2
  Constant24/1 -> Mult/1
  AddSub1/1 -> Mux4/3
  Mult/1 -> AddSub1/2
  [buffer_we] -> Gateway Out2/1
  [ant_number] -> Gateway Out3/1
  [buffer_addr] -> Gateway Out4/1
  [valid] -> Gateway Out5/1
  [block_step] -> Gateway Out6/1
  [ant_in_block] -> Gateway Out7/1
  [ant_in_block] -> "select_antenna "/2(antenna_in_block)
  transpose/1(sync_out) -> "select_antenna "/1(sync_in)
  "select_antenna "/1(sync_out) -> bus-convert-16b/1(sync_in)
  Delay3/1 -> [valid]
  [valid] -> Delay11/1
  bus-convert-16b/1(sync_out) -> Delay13/1, count-words/1
  Delay13/1 -> [final_valid]
  Delay14/1 -> eof/1, Counter2/1, Logical3/2
  Gateway Out7/1 -> Scope5/1
  Gateway Out6/1 -> Scope4/1
  Gateway Out5/1 -> Scope3/1
  Gateway Out4/1 -> Scope2/1
  Gateway Out3/1 -> Scope1/1
  Gateway Out2/1 -> Scope/1
  Gateway Out9/1 -> Scope7/1
  bus_expand3/1(msb_out16) -> Gateway Out9/1
  Gateway Out10/1 -> Scope8/1
  bus_expand3/2(out15) -> Gateway Out10/1
  Gateway Out11/1 -> Scope9/1
  bus_expand3/3(out14) -> Gateway Out11/1
  Gateway Out12/1 -> Scope10/1
  bus_expand3/4(out13) -> Gateway Out12/1
  Gateway Out15/1 -> Scope11/1
  Gateway Out14/1 -> Scope14/1
  Gateway Out13/1 -> Scope13/1
  Gateway Out16/1 -> Scope12/1
  bus_expand3/8(out9) -> Gateway Out15/1
  bus_expand3/5(out12) -> Gateway Out16/1
  bus_expand3/6(out11) -> Gateway Out13/1
  bus_expand3/7(out10) -> Gateway Out14/1
  Gateway Out23/1 -> Scope18/1
  Gateway Out20/1 -> Scope19/1
  Gateway Out21/1 -> Scope20/1
  Gateway Out22/1 -> Scope17/1
  Gateway Out19/1 -> Scope16/1
  Gateway Out18/1 -> Scope23/1
  Gateway Out17/1 -> Scope22/1
  Gateway Out24/1 -> Scope21/1
  bus_expand3/16(lsb_out1) -> Gateway Out22/1
  bus_expand3/15(out2) -> Gateway Out21/1
  bus_expand3/14(out3) -> Gateway Out20/1
  bus_expand3/13(out4) -> Gateway Out23/1
  bus_expand3/12(out5) -> Gateway Out19/1
  bus_expand3/11(out6) -> Gateway Out18/1
  bus_expand3/10(out7) -> Gateway Out17/1
  bus_expand3/9(out8) -> Gateway Out24/1
  [final_valid] -> Gateway Out25/1
  [eof] -> Gateway Out26/1
  Gateway Out25/1 -> Scope24/1
  Gateway Out26/1 -> Scope25/1
  Gateway Out27/1 -> Scope26/1
  [cr_40g_rst] -> eth40g_rst_out/1
  [readout_done_rst] -> count-to-8/1
  Relational4/1 -> edge_detect2/1(in), Gateway Out32/1
  edge_detect4/1(out) -> [eof]
  Gateway Out8/1 -> Scope6/1
  Constant/1 -> bus_create4/2(in2)
  Gateway Out28/1 -> Scope27/1
  [readout_done] -> Gateway Out28/1
  Gateway Out30/1 -> Scope29/1
  Gateway Out31/1 -> Scope30/1
  [readout_done_rst] -> count-limited-counter/3(rst)
  edge_detect1/1(out) -> pulse_ext/1(in), [readout_done]
  pulse_ext/1(out) -> [readout_done_rst]
  Constant3/1 -> Relational4/1
  edge_detect2/1(out) -> antenna_counter/2, Gateway Out33/1
  [packetwait] -> Relational2/2
  Delay16/1 -> buffer_addr/1, count-to-8/2, Gateway Out27/1
  Constant25/1 -> Relational7/1
  Relational7/1 -> edge_detect3/1(in)
  Relational5/1 -> edge_detect4/1(in)
  Constant4/1 -> Relational5/1
  [readout_done] -> "readout_done "/1
  Relational1/1 -> edge_detect1/1(in)
  Constant1/1 -> Relational1/1
  Gateway Out29/1 -> Scope28/1
  Gateway Out32/1 -> Scope31/1
  Gateway Out33/1 -> Scope32/1
  [readout_done_rst] -> Gateway Out34/1, antenna_counter/1
  Gateway Out34/1 -> Scope33/1
  [buffer_addr] -> Delay4/1
  AddSub3/1 -> Dual Port RAM/4
  [buffer_addr] -> AddSub3/1
  Constant26/1 -> AddSub3/2
  AddSub2/1 -> Dual Port RAM1/4
  [buffer_addr] -> AddSub2/1
  Constant2/1 -> AddSub2/2
  Constant27/1 -> AddSub4/2
  [buffer_addr] -> AddSub4/1
  AddSub4/1 -> Dual Port RAM2/4
  [buffer_addr] -> AddSub5/1
  Constant29/1 -> AddSub5/2
  Constant30/1 -> AddSub6/2
  [buffer_addr] -> AddSub6/1
  [buffer_addr] -> AddSub7/1
  Constant31/1 -> AddSub7/2
  Constant32/1 -> AddSub8/2
  [buffer_addr] -> AddSub8/1
  [buffer_addr] -> AddSub9/1
  Constant34/1 -> AddSub9/2
  AddSub9/1 -> Dual Port RAM7/4
  AddSub8/1 -> Dual Port RAM6/4
  AddSub7/1 -> Dual Port RAM5/4
  AddSub6/1 -> Dual Port RAM4/4
  AddSub5/1 -> Dual Port RAM3/4
  Mux2/1 -> transpose/2(data_in)
  Delay17/1 -> Mux1/3
  Delay24/1 -> bus-convert-16b/2(data_in)
  transpose/2(data_out) -> Delay24/1
  [telescopetime] -> tt_counter/2
  [packetizer_sync] -> tt_counter/1
  delay_buffer/1 -> delay_bram_prog2/2, delay_bram_prog1/2
  data_in/1 -> delay_bram_prog1/1
  delay_bram_prog1/1 -> bus_expand1/1(bus_in)
  tt_counter/1 -> delay_bram_prog2/1
  delay_bram_prog2/1 -> Single Port RAM1/2

== system snap2_f_200msps_64i_4096c/cosmic_ray/bus_create ==
  in1 : Inport
  in2 : Inport  Port=2
  in3 : Inport  Port=3
  in4 : Inport  Port=4
  in5 : Inport  Port=5
  in6 : Inport  Port=6
  in7 : Inport  Port=7
  in8 : Inport  Port=8
  in9 : Inport  Port=9
  in10 : Inport  Port=10
  concatenate : xbsIndex_r4/Concat  num_inputs=10  dbl_ovrd=off  block_type=concat
  reinterpret{1..10} (10 alike) : xbsIndex_r4/Reinterpret  force_arith_type=on  arith_type=Unsigned  force_bin_pt=on  bin_pt=0  block_type=reinterpret
      reinterpret1 settings: infoedit="Changes signal type without altering the binary representation.   You can changed the signal between signed and unsigned, and relocate the binary point.<br><br>Hardware notes: In hardware this block costs nothing.<br><br>Example:  Suppose the input is 6 bits wide, signed, with 2 fractional bits, and the output is forced to unsigned with 0 fractional bits.  Then an input of -2.0 (1110.00 in binary 2's complement) becomes an output of 56 (111000 in binary)."
      reinterpret2 settings: infoedit="Changes signal type without altering the binary representation.   You can changed the signal between signed and unsigned, and relocate the binary point.<br><br>Hardware notes: In hardware this block costs nothing.<br><br>Example:  Suppose the input is 6 bits wide, signed, with 2 fractional bits, and the output is forced to unsigned with 0 fractional bits.  Then an input of -2.0 (1110.00 in binary 2's complement) becomes an output of 56 (111000 in binary)."
  bus_out : Outport
  wires:
  concatenate/1 -> bus_out/1
  in1/1 -> reinterpret1/1
  reinterpret1/1 -> concatenate/1
  in2/1 -> reinterpret2/1
  reinterpret2/1 -> concatenate/2
  in3/1 -> reinterpret3/1
  reinterpret3/1 -> concatenate/3
  in4/1 -> reinterpret4/1
  reinterpret4/1 -> concatenate/4
  in5/1 -> reinterpret5/1
  reinterpret5/1 -> concatenate/5
  in6/1 -> reinterpret6/1
  reinterpret6/1 -> concatenate/6
  in7/1 -> reinterpret7/1
  reinterpret7/1 -> concatenate/7
  in8/1 -> reinterpret8/1
  reinterpret8/1 -> concatenate/8
  in9/1 -> reinterpret9/1
  reinterpret9/1 -> concatenate/9
  in10/1 -> reinterpret10/1
  reinterpret10/1 -> concatenate/10

== system snap2_f_200msps_64i_4096c/cosmic_ray/bus_create4 ==
  in1 : Inport
  in2 : Inport  Port=2
  concatenate : xbsIndex_r4/Concat  num_inputs=2  dbl_ovrd=off  block_type=concat
  reinterpret1 : xbsIndex_r4/Reinterpret  force_arith_type=on  arith_type=Unsigned  force_bin_pt=on  bin_pt=0  block_type=reinterpret
      settings: infoedit="Changes signal type without altering the binary representation.   You can changed the signal between signed and unsigned, and relocate the binary point.<br><br>Hardware notes: In hardware this block costs nothing.<br><br>Example:  Suppose the input is 6 bits wide, signed, with 2 fractional bits, and the output is forced to unsigned with 0 fractional bits.  Then an input of -2.0 (1110.00 in binary 2's complement) becomes an output of 56 (111000 in binary)."
  reinterpret2 : xbsIndex_r4/Reinterpret  force_arith_type=on  arith_type=Unsigned  force_bin_pt=on  bin_pt=0  block_type=reinterpret
      settings: infoedit="Changes signal type without altering the binary representation.   You can changed the signal between signed and unsigned, and relocate the binary point.<br><br>Hardware notes: In hardware this block costs nothing.<br><br>Example:  Suppose the input is 6 bits wide, signed, with 2 fractional bits, and the output is forced to unsigned with 0 fractional bits.  Then an input of -2.0 (1110.00 in binary 2's complement) becomes an output of 56 (111000 in binary)."
  bus_out : Outport
  wires:
  concatenate/1 -> bus_out/1
  in1/1 -> reinterpret1/1
  reinterpret1/1 -> concatenate/1
  in2/1 -> reinterpret2/1
  reinterpret2/1 -> concatenate/2
